simulink model "feng_ct"  (R2016b)
settings: Solver=VariableStepAuto  StartTime=0.0  StopTime=5000  RelTol=1e-3  EnableMultiTasking=on
undefined symbols (not defined in the file or in its folder): fft_stages, output_len_bits, xengbits
undefined symbols (not defined in the file): input_bits, total_bits, total_bits2
libraries: xbsIndex_r4 x10571, casper_library_misc x48, casper_library_scopes x9, xps_library x2
(part 11 of 81)

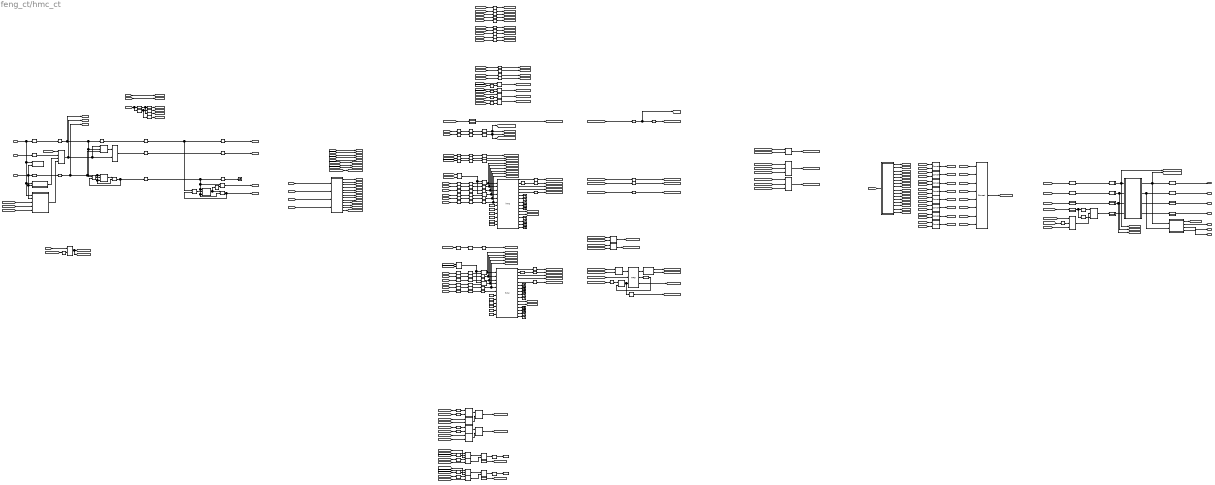
== system feng_ct/hmc_ct ==
  note: Double buffer the data to form output packets
  note: Eight parallel channels.
  note: TVG
  note: Write two successive words together.
  note: Sync debugging - did we get two syncs
      | so close we weren't even reading out yet?
  note: Check for _en sync and bank errors
  note: HMC
  in_sync : Inport
  in_dv : Inport  Port=2
  in_d128 : Inport  Port=3
  Assertion : Assertion
  Assertion1 : Assertion
  Concat{3..10,12} (9 alike) : xbsIndex_r4/Concat  num_inputs=2  dbl_ovrd=off  block_type=concat
  Concat11 : xbsIndex_r4/Concat  num_inputs=8  dbl_ovrd=off  block_type=concat
  Concat13 : xbsIndex_r4/Concat  num_inputs=3  dbl_ovrd=off  block_type=concat
  Constant{,3,6,9} (4 alike) : xbsIndex_r4/Constant  const=0  gui_display_data_type=Boolean  arith_type=Boolean  n_bits=16  bin_pt=14  preci_type=Single  exp_width=8  frac_width=24  explicit_period=on  period=1  equ=P=C  opselect=C  inp2=PCIN>>17  opr=+  inp1=P  carry=CIN  dbl_ovrd=off  block_type=constant
  Constant{1,4,7,10} (4 alike) : xbsIndex_r4/Constant  const=0  gui_display_data_type=Fixed-point  arith_type=Unsigned  n_bits=27  bin_pt=0  preci_type=Single  exp_width=8  frac_width=24  explicit_period=on  period=1  equ=P=C  opselect=C  inp2=PCIN>>17  opr=+  inp1=P  carry=CIN  dbl_ovrd=off  block_type=constant
  Constant11 : xbsIndex_r4/Constant  const=0  gui_display_data_type=Fixed-point  arith_type=Unsigned  n_bits=9  bin_pt=0  preci_type=Single  exp_width=8  frac_width=24  explicit_period=on  period=1  equ=P=C  opselect=C  inp2=PCIN>>17  opr=+  inp1=P  carry=CIN  dbl_ovrd=off  block_type=constant
  Constant12 : xbsIndex_r4/Constant  const=0  gui_display_data_type=Boolean  arith_type=Boolean  n_bits=9  bin_pt=0  preci_type=Single  exp_width=8  frac_width=24  explicit_period=on  period=1  equ=P=C  opselect=C  inp2=PCIN>>17  opr=+  inp1=P  carry=CIN  dbl_ovrd=off  block_type=constant
  Constant13 : xbsIndex_r4/Constant  const=0  gui_display_data_type=Boolean  arith_type=Boolean  n_bits=9  bin_pt=0  preci_type=Single  exp_width=8  frac_width=24  explicit_period=on  period=1  equ=P=C  opselect=C  inp2=PCIN>>17  opr=+  inp1=P  carry=CIN  dbl_ovrd=off  block_type=constant
  Constant2 : xbsIndex_r4/Constant  const=0  gui_display_data_type=Fixed-point  arith_type=Unsigned  n_bits=256  bin_pt=0  preci_type=Single  exp_width=8  frac_width=24  explicit_period=on  period=1  equ=P=C  opselect=C  inp2=PCIN>>17  opr=+  inp1=P  carry=CIN  dbl_ovrd=off  block_type=constant
  Constant5 : xbsIndex_r4/Constant  const=0  gui_display_data_type=Fixed-point  arith_type=Unsigned  n_bits=9  bin_pt=0  preci_type=Single  exp_width=8  frac_width=24  explicit_period=on  period=1  equ=P=C  opselect=C  inp2=PCIN>>17  opr=+  inp1=P  carry=CIN  dbl_ovrd=off  block_type=constant
  Constant8 : xbsIndex_r4/Constant  const=0  gui_display_data_type=Fixed-point  arith_type=Unsigned  n_bits=256  bin_pt=0  preci_type=Single  exp_width=8  frac_width=24  explicit_period=on  period=1  equ=P=C  opselect=C  inp2=PCIN>>17  opr=+  inp1=P  carry=CIN  dbl_ovrd=off  block_type=constant
  Delay{,1..2,4..13,16..19,21..23,25..27,30..32,41,43..50,52..53,56..58,61..62,66..69,72,74,76..92} (65 alike) : xbsIndex_r4/Delay  rst=off  infoeditControl=Selection of Reset will increase slice count due to use of real FFs and instead of SRLs  en=off  latency=1  reg_retiming=off  dbl_ovrd=off  block_type=delay
      settings: infoedit=Hardware notes: A delay line is a chain, each link of which is an SRL16 or SRL32 followed by a flip-flop.
  Delay{14..15,35,39,42,93} (6 alike) : xbsIndex_r4/Delay  rst=off  infoeditControl=Selection of Reset will increase slice count due to use of real FFs and instead of SRLs  en=off  latency=2  reg_retiming=off  dbl_ovrd=off  block_type=delay
      settings: infoedit=Hardware notes: A delay line is a chain, each link of which is an SRL16 or SRL32 followed by a flip-flop.
  Delay{3,20,24,28..29,37..38,40,55,59,63,70..71,73} (14 alike) : xbsIndex_r4/Delay  rst=off  infoeditControl=Selection of Reset will increase slice count due to use of real FFs and instead of SRLs  en=off  latency=5  reg_retiming=off  dbl_ovrd=off  block_type=delay
      settings: infoedit=Hardware notes: A delay line is a chain, each link of which is an SRL16 or SRL32 followed by a flip-flop.
  Delay33 : xbsIndex_r4/Delay  rst=off  infoeditControl=Selection of Reset will increase slice count due to use of real FFs and instead of SRLs  en=off  latency=4  reg_retiming=off  dbl_ovrd=off  block_type=delay
      settings: infoedit=Hardware notes: A delay line is a chain, each link of which is an SRL16 or SRL32 followed by a flip-flop.
  Delay34 : xbsIndex_r4/Delay  rst=off  infoeditControl=Selection of Reset will increase slice count due to use of real FFs and instead of SRLs  en=off  latency=4  reg_retiming=off  dbl_ovrd=off  block_type=delay
      settings: infoedit=Hardware notes: A delay line is a chain, each link of which is an SRL16 or SRL32 followed by a flip-flop.
  Delay36 : xbsIndex_r4/Delay  rst=off  infoeditControl=Selection of Reset will increase slice count due to use of real FFs and instead of SRLs  en=off  latency=4  reg_retiming=off  dbl_ovrd=off  block_type=delay
      settings: infoedit=Hardware notes: A delay line is a chain, each link of which is an SRL16 or SRL32 followed by a flip-flop.
  Inverter{,1..11,15..16} (14 alike) : xbsIndex_r4/Inverter  en=off  latency=0  dbl_ovrd=off  block_type=inv
  Logical{,3,8,19,21,29..31} (8 alike) : xbsIndex_r4/Logical  logical_function=AND  inputs=2  en=off  latency=0  precision=Full  arith_type=Unsigned  n_bits=16  bin_pt=0  align_bp=on  dbl_ovrd=off  block_type=logical
  Logical1 : xbsIndex_r4/Logical  logical_function=AND  inputs=2  en=off  latency=1  precision=User Defined  arith_type=Boolean  n_bits=1  bin_pt=0  align_bp=on  dbl_ovrd=off  block_type=logical
  Logical{2,9..10,20} (4 alike) : xbsIndex_r4/Logical  logical_function=OR  inputs=2  en=off  latency=0  precision=Full  arith_type=Unsigned  n_bits=16  bin_pt=0  align_bp=on  dbl_ovrd=off  block_type=logical
  Logical{5,7,11,13,17..18,22,28} (8 alike) : xbsIndex_r4/Logical  logical_function=AND  inputs=2  en=off  latency=5  precision=Full  arith_type=Unsigned  n_bits=16  bin_pt=0  align_bp=on  dbl_ovrd=off  block_type=logical
  Logical{4,12,16,26} (4 alike) : xbsIndex_r4/Logical  logical_function=AND  inputs=2  en=off  latency=1  precision=Full  arith_type=Unsigned  n_bits=16  bin_pt=0  align_bp=on  dbl_ovrd=off  block_type=logical
  Logical14 : xbsIndex_r4/Logical  logical_function=OR  inputs=2  en=off  latency=5  precision=Full  arith_type=Unsigned  n_bits=16  bin_pt=0  align_bp=on  dbl_ovrd=off  block_type=logical
  Logical15 : xbsIndex_r4/Logical  logical_function=AND  inputs=2  en=off  latency=2  precision=Full  arith_type=Unsigned  n_bits=16  bin_pt=0  align_bp=on  dbl_ovrd=off  block_type=logical
  Logical23 : xbsIndex_r4/Logical  logical_function=OR  inputs=2  en=off  latency=5  precision=Full  arith_type=Unsigned  n_bits=16  bin_pt=0  align_bp=on  dbl_ovrd=off  block_type=logical
  Logical24 : xbsIndex_r4/Logical  logical_function=AND  inputs=3  en=off  latency=5  precision=Full  arith_type=Unsigned  n_bits=16  bin_pt=0  align_bp=on  dbl_ovrd=off  block_type=logical
  Logical25 : xbsIndex_r4/Logical  logical_function=AND  inputs=2  en=off  latency=1  precision=User Defined  arith_type=Boolean  n_bits=1  bin_pt=0  align_bp=on  dbl_ovrd=off  block_type=logical
  Logical32 : xbsIndex_r4/Logical  logical_function=OR  inputs=2  en=off  latency=2  precision=Full  arith_type=Unsigned  n_bits=16  bin_pt=0  align_bp=on  dbl_ovrd=off  block_type=logical
  Logical6 : xbsIndex_r4/Logical  logical_function=AND  inputs=3  en=off  latency=5  precision=Full  arith_type=Unsigned  n_bits=16  bin_pt=0  align_bp=on  dbl_ovrd=off  block_type=logical
  Mux : xbsIndex_r4/Mux  inputs=2  en=off  latency=2  precision=Full  arith_type=Unsigned  n_bits=16  bin_pt=14  quantization=Truncate  overflow=Wrap  dbl_ovrd=off  block_type=mux
  Mux1 : xbsIndex_r4/Mux  inputs=2  en=off  latency=2  precision=Full  arith_type=Unsigned  n_bits=16  bin_pt=14  quantization=Truncate  overflow=Wrap  dbl_ovrd=off  block_type=mux
  Mux2 : xbsIndex_r4/Mux  inputs=2  en=off  latency=2  precision=Full  arith_type=Unsigned  n_bits=16  bin_pt=14  quantization=Truncate  overflow=Wrap  dbl_ovrd=off  block_type=mux
  Mux3 : xbsIndex_r4/Mux  inputs=3  en=off  latency=2  precision=Full  arith_type=Unsigned  n_bits=16  bin_pt=14  quantization=Truncate  overflow=Wrap  dbl_ovrd=off  block_type=mux
  Register : xbsIndex_r4/Register  init=0  rst=on  en=on  dbl_ovrd=off  block_type=register
  Register1 : xbsIndex_r4/Register  init=0  rst=on  en=on  dbl_ovrd=off  block_type=register
  Slice{8..9,12..13} (4 alike) : xbsIndex_r4/Slice  nbits=1  boolean_output=on  mode=Lower Bit Location + Width  bit1=0  base1=MSB of Input  bit0=input_len_bits - 2 + output_len_bits  base0=LSB of Input  dbl_ovrd=off  block_type=slice
  Terminator{,1..18} (19 alike) : Terminator
  bank2 : xbsIndex_r4/Slice  nbits=12  boolean_output=off  mode=Upper Bit Location + Width  bit1=-4  base1=MSB of Input  bit0=128  base0=LSB of Input  dbl_ovrd=off  block_type=slice
  bank3 : xbsIndex_r4/Slice  nbits=12  boolean_output=off  mode=Upper Bit Location + Width  bit1=-4  base1=MSB of Input  bit0=128  base0=LSB of Input  dbl_ovrd=off  block_type=slice
  bank4 : xbsIndex_r4/Slice  nbits=128  boolean_output=off  mode=Lower Bit Location + Width  bit1=0  base1=MSB of Input  bit0=128  base0=LSB of Input  dbl_ovrd=off  block_type=slice
  bank5 : xbsIndex_r4/Slice  nbits=128  boolean_output=off  mode=Lower Bit Location + Width  bit1=0  base1=MSB of Input  bit0=0  base0=LSB of Input  dbl_ovrd=off  block_type=slice
  bank6 : xbsIndex_r4/Slice  nbits=12  boolean_output=on  mode=Upper Bit Location + Width  bit1=0  base1=MSB of Input  bit0=128  base0=LSB of Input  dbl_ovrd=off  block_type=slice
  bank7 : xbsIndex_r4/Slice  nbits=12  boolean_output=on  mode=Upper Bit Location + Width  bit1=0  base1=MSB of Input  bit0=128  base0=LSB of Input  dbl_ovrd=off  block_type=slice
  bus_create1 : Subsystem  AncestorBlock=casper_library_flow_control/bus_create  mask(bus_create){inputNum=2}
      mask prompts: inputNum "Number of inputs:"
      mask init:
      | bus_create_init(gcb,...
      |     'inputNum', inputNum);
  bus_expand1 : Subsystem  AncestorBlock=casper_library_flow_control/bus_expand  mask(bus_expand){mode=divisions of equal size, outputNum=16, outputWidth=16, outputBinaryPt=0, outputArithmeticType=0, show_format=off, outputToWorkspace=off, variablePrefix=out, outputToModelAsWell=on}
      mask prompts: outputNum "Number of outputs:"; outputWidth "Output width:"; outputBinaryPt "Output binary point position:"; outputArithmeticType "Output arithmetic type (ufix=0, fix=1, bool=2):"; show_format "Print format string?"; outputToWorkspace "Output to workspace?"; variablePrefix "Variable name prefix:"; outputToModelAsWell "Output to model as well?"
      mask help:
      | Expands a 'bus' made using a bus_create or Xilinx
      | concat block.
      | The input will be divided into the specified number
      | of outputs with the specified arithmetic types.
      | Divisions are made from most significant bit.
      mask init: same as feng_ct/bus_expand1
      settings: AttributesFormatString=16 outputs
      mask TypeOptions mode: divisions of equal size | divisions of arbitrary size
      mask Callback mode: bus_expand_callback();
      mask Callback outputWidth: bus_expand_callback();
      mask Callback outputToWorkspace: bus_expand_callback();
  bus_expand2 : Subsystem  AncestorBlock=casper_library_flow_control/bus_expand  mask(bus_expand){mode=divisions of arbitrary size, outputNum=1, outputWidth=[256 9], outputBinaryPt=0, outputArithmeticType=0, show_format=on, outputToWorkspace=off, variablePrefix=out, outputToModelAsWell=on}
      mask prompts: outputNum "Number of outputs:"; outputWidth "Output width [msb ... lsb]:"; outputBinaryPt "Output binary point position [msb ... lsb]:"; outputArithmeticType "Output arithmetic type (ufix=0, fix=1, bool=2) [msb ... lsb]:"; show_format "Print format string?"; outputToWorkspace "Output to workspace?"; variablePrefix "Variable name prefix:"; outputToModelAsWell "Output to model as well?"
      mask help:
      | Expands a 'bus' made using a bus_create or Xilinx
      | concat block.
      | The input will be divided into the specified number
      | of outputs with the specified arithmetic types.
      | Divisions are made from most significant bit.
      mask init: same as feng_ct/bus_expand1
      settings: AttributesFormatString=2 outputs: uf256.0,uf9.0,
      mask TypeOptions mode: divisions of equal size | divisions of arbitrary size
      mask Callback mode: bus_expand_callback();
      mask Callback outputWidth: bus_expand_callback();
      mask Callback outputToWorkspace: bus_expand_callback();
  convert_rd_en1 : xbsIndex_r4/Convert  gui_display_data_type=Boolean  arith_type=Boolean  n_bits=128  bin_pt=0  float_type=Single  exp_bits=8  fraction_bits=24  quantization=Truncate  overflow=Wrap  en=off  latency=0  pipeline=off  dbl_ovrd=off  block_type=convert
      settings: xl_area=[0, 0, 0, 0, 0, 0, 0]
  convert_rd_en4 : xbsIndex_r4/Convert  gui_display_data_type=Boolean  arith_type=Boolean  n_bits=128  bin_pt=0  float_type=Single  exp_bits=8  fraction_bits=24  quantization=Truncate  overflow=Wrap  en=off  latency=0  pipeline=off  dbl_ovrd=off  block_type=convert
      settings: xl_area=[0, 0, 0, 0, 0, 0, 0]
  d1_fifo : xbsIndex_r4/FIFO  mem_type=Distributed RAM  performance_options=Standard_FIFO  embedded_registers=off  depth=16  percent_nbits=1  rst=off  rst_latency=1  en=off  use_dcount=off  use_percent_full_port=off  use_almost_empty=off  almost_empty_thresh=2  use_almost_full=off  almost_full_thresh=14  explicit_period=off  dbl_ovrd=off  block_type=fifo
  edge_detect1 : Subsystem  AncestorBlock=casper_library_misc/edge_detect  mask(edge_detect){edge=Rising, polarity=Active High, x_in=[0 0.08 0.08 0.16 0.16 0.24 0.24 0.32 0.32 0.4], y_in=[-1 -1  1  1  1  1  1  1  1  1], x_out=[0.6 0.68 0.68 0.76 0.76 0.84 0.84 0.92 0.92 1], y_out=[-1 -1  1  1 -1 -1 -1 -1 -1 -1]}
      mask prompts: edge "Edge Type"; polarity "Output Polarity"; x_in "Input X Positions"; y_in "Input Y Positions"; x_out "Output X Positions"; y_out "Output Y Positions"
      mask help: Output is active for one-cycle after each edge of the specified type (i.e. rising, falling or both).
      mask init: same as feng_ct/edge_detect1
      settings: AttributesFormatString=|
      | rising edges
      | active high
      mask Help: Output is active for one-cycle after each edge of the specified type (i.e. rising, falling, or both).  Latency is zero.
      mask TypeOptions edge: Rising | Falling | Both
      mask TypeOptions polarity: Active High | Active Low
      mask Display:
      | plot(x_in_num,0.5+y_in_num*0.2);
      | plot(x_out_num,0.5+y_out_num*0.2);
  gen_freq_calc : Subsystem  mask{pkt_len_bits=5, lat=3}
      mask prompts: pkt_len_bits "Packet length bits"; lat "Latency"
      mask init:
      | display_string = sprintf('latency=%i', 7 * lat);
      | set_param(gcb, 'AttributesFormatString', display_string);
      settings: AttributesFormatString=latency=21
  hmc : xps_library/hmc  Tag=xps:hmc  mez=0  sim_depth=(input_len_bits-1) + output_len_bits + 1  sim_latency=5  sim_rand=on
  hmc1 : xps_library/hmc  Tag=xps:hmc  mez=1  sim_depth=(input_len_bits-1) + output_len_bits + 1  sim_latency=5  sim_rand=on
  hmc_addr_gen : Subsystem  mask{input_len_bits=input_len_bits - 1}
      mask prompts: input_len_bits "Input vector bits"
  obuf : Subsystem  mask{output_vec_bits=output_len_bits, pkt_buffer_latency=10, omux_latency=15}
      mask prompts: output_vec_bits "CT output vector bits"; pkt_buffer_latency "Output buffer latency"; omux_latency "Output mux latency"
  prev_word : xbsIndex_r4/Register  init=0  rst=on  en=on  dbl_ovrd=off  block_type=register
  spectrum_ctr2 : xbsIndex_r4/Slice  nbits=256 - (32 + 9)  boolean_output=off  mode=Lower Bit Location + Width  bit1=-1  base1=MSB of Input  bit0=32 + 9  base0=LSB of Input  dbl_ovrd=off  block_type=slice
  spectrum_ctr3 : xbsIndex_r4/Slice  nbits=32  boolean_output=off  mode=Lower Bit Location + Width  bit1=-1  base1=MSB of Input  bit0=0  base0=LSB of Input  dbl_ovrd=off  block_type=slice
  spectrum_ctr4 : xbsIndex_r4/Slice  nbits=9  boolean_output=off  mode=Lower Bit Location + Width  bit1=-1  base1=MSB of Input  bit0=32  base0=LSB of Input  dbl_ovrd=off  block_type=slice
  tvg_data_gen : Subsystem
  tvg_data_gen_oneshot : Subsystem
      mask Display:
      | color('red');
      | disp('ONE SHOT!!');
      | % color('green');
      | % port_label('input', 1, 'dv')
      | % color('red');
      | % port_label('output', 1, 'err')
  tvg_data_tone_gen : Subsystem
  we_delay1 : Subsystem  AncestorBlock=casper_library_delays/pipeline  mask(pipeline){latency=2}
      mask help:
      | An explicitly laid-out delay line to avoid mapping to SRL16s
      | for use in pipelining to help achieve timing closure.
      mask init:
      | pipeline_init(gcb,'latency',latency);
      settings: AttributesFormatString=Latency = %<latency>
      mask Display:
      | port_label('input', 1, 'd');
      | port_label('output', 1, 'q');
      | disp(['Z^-', num2str(latency)]);
  we_delay10 : Subsystem  AncestorBlock=casper_library_delays/pipeline  mask(pipeline){latency=21}
      mask help:
      | An explicitly laid-out delay line to avoid mapping to SRL16s
      | for use in pipelining to help achieve timing closure.
      mask init:
      | pipeline_init(gcb,'latency',latency);
      settings: AttributesFormatString=Latency = %<latency>
      mask Display:
      | port_label('input', 1, 'd');
      | port_label('output', 1, 'q');
      | disp(['Z^-', num2str(latency)]);
  we_delay11 : Subsystem  AncestorBlock=casper_library_delays/pipeline  mask(pipeline){latency=2}
      mask help:
      | An explicitly laid-out delay line to avoid mapping to SRL16s
      | for use in pipelining to help achieve timing closure.
      mask init:
      | pipeline_init(gcb,'latency',latency);
      settings: AttributesFormatString=Latency = %<latency>
      mask Display:
      | port_label('input', 1, 'd');
      | port_label('output', 1, 'q');
      | disp(['Z^-', num2str(latency)]);
  we_delay12 : Subsystem  AncestorBlock=casper_library_delays/pipeline  mask(pipeline){latency=21}
      mask help:
      | An explicitly laid-out delay line to avoid mapping to SRL16s
      | for use in pipelining to help achieve timing closure.
      mask init:
      | pipeline_init(gcb,'latency',latency);
      settings: AttributesFormatString=Latency = %<latency>
      mask Display:
      | port_label('input', 1, 'd');
      | port_label('output', 1, 'q');
      | disp(['Z^-', num2str(latency)]);
  we_delay2 : Subsystem  AncestorBlock=casper_library_delays/pipeline  mask(pipeline){latency=2}
      mask help:
      | An explicitly laid-out delay line to avoid mapping to SRL16s
      | for use in pipelining to help achieve timing closure.
      mask init:
      | pipeline_init(gcb,'latency',latency);
      settings: AttributesFormatString=Latency = %<latency>
      mask Display:
      | port_label('input', 1, 'd');
      | port_label('output', 1, 'q');
      | disp(['Z^-', num2str(latency)]);
  we_delay3 : Subsystem  AncestorBlock=casper_library_delays/pipeline  mask(pipeline){latency=2}
      mask help:
      | An explicitly laid-out delay line to avoid mapping to SRL16s
      | for use in pipelining to help achieve timing closure.
      mask init:
      | pipeline_init(gcb,'latency',latency);
      settings: AttributesFormatString=Latency = %<latency>
      mask Display:
      | port_label('input', 1, 'd');
      | port_label('output', 1, 'q');
      | disp(['Z^-', num2str(latency)]);
  we_delay4 : Subsystem  AncestorBlock=casper_library_delays/pipeline  mask(pipeline){latency=2}
      mask help:
      | An explicitly laid-out delay line to avoid mapping to SRL16s
      | for use in pipelining to help achieve timing closure.
      mask init:
      | pipeline_init(gcb,'latency',latency);
      settings: AttributesFormatString=Latency = %<latency>
      mask Display:
      | port_label('input', 1, 'd');
      | port_label('output', 1, 'q');
      | disp(['Z^-', num2str(latency)]);
  we_delay5 : Subsystem  AncestorBlock=casper_library_delays/pipeline  mask(pipeline){latency=2}
      mask help:
      | An explicitly laid-out delay line to avoid mapping to SRL16s
      | for use in pipelining to help achieve timing closure.
      mask init:
      | pipeline_init(gcb,'latency',latency);
      settings: AttributesFormatString=Latency = %<latency>
      mask Display:
      | port_label('input', 1, 'd');
      | port_label('output', 1, 'q');
      | disp(['Z^-', num2str(latency)]);
  we_delay6 : Subsystem  AncestorBlock=casper_library_delays/pipeline  mask(pipeline){latency=2}
      mask help:
      | An explicitly laid-out delay line to avoid mapping to SRL16s
      | for use in pipelining to help achieve timing closure.
      mask init:
      | pipeline_init(gcb,'latency',latency);
      settings: AttributesFormatString=Latency = %<latency>
      mask Display:
      | port_label('input', 1, 'd');
      | port_label('output', 1, 'q');
      | disp(['Z^-', num2str(latency)]);
  we_delay7 : Subsystem  AncestorBlock=casper_library_delays/pipeline  mask(pipeline){latency=2}
      mask help:
      | An explicitly laid-out delay line to avoid mapping to SRL16s
      | for use in pipelining to help achieve timing closure.
      mask init:
      | pipeline_init(gcb,'latency',latency);
      settings: AttributesFormatString=Latency = %<latency>
      mask Display:
      | port_label('input', 1, 'd');
      | port_label('output', 1, 'q');
      | disp(['Z^-', num2str(latency)]);
  we_delay8 : Subsystem  AncestorBlock=casper_library_delays/pipeline  mask(pipeline){latency=21}
      mask help:
      | An explicitly laid-out delay line to avoid mapping to SRL16s
      | for use in pipelining to help achieve timing closure.
      mask init:
      | pipeline_init(gcb,'latency',latency);
      settings: AttributesFormatString=Latency = %<latency>
      mask Display:
      | port_label('input', 1, 'd');
      | port_label('output', 1, 'q');
      | disp(['Z^-', num2str(latency)]);
  we_delay9 : Subsystem  AncestorBlock=casper_library_delays/pipeline  mask(pipeline){latency=21}
      mask help:
      | An explicitly laid-out delay line to avoid mapping to SRL16s
      | for use in pipelining to help achieve timing closure.
      mask init:
      | pipeline_init(gcb,'latency',latency);
      settings: AttributesFormatString=Latency = %<latency>
      mask Display:
      | port_label('input', 1, 'd');
      | port_label('output', 1, 'q');
      | disp(['Z^-', num2str(latency)]);
  out_sync : Outport
  out_dv : Outport  Port=2
  out_d256 : Outport  Port=3
  pkt_start : Outport  Port=4
  freq_id : Outport  Port=5
  x_index : Outport  Port=6
  x_pkt_index : Outport  Port=7
  tag scope: ct_bank_error_g0=global, ct_bank_error_g1=global, ct_en_sync_error_g0=global, ct_en_sync_error_g1=global, ct_in_d0_g=global, ct_in_d0_msb_g=global, ct_in_d1_g=global, ct_in_d1_msb_g=global, ct_in_dv_g=global, ct_in_sync_g=global, cthmc_sync_err_g0=global, cthmc_sync_err_g1=global, hmc_d256_g0=global, hmc_d256_g1=global, hmc_dv_clash_g=global, hmc_dv_fixed_clash_g=global, hmc_dv_g0=global, hmc_dv_g1=global, hmc_err_rdrdy_g0=global, hmc_err_rdrdy_g1=global, hmc_err_wrrdy_g0=global, hmc_err_wrrdy_g1=global, hmc_fifo_full_g=global, hmc_init_done_g0=global, hmc_init_done_g1=global, hmc_postokay_g0=global, hmc_postokay_g1=global, hmc_rd_rdy_g0=global, hmc_rd_rdy_g1=global, hmc_sync_g=global, hmc_tag_g0=global, hmc_tag_g1=global, hmc_wr_rdy_g0=global, hmc_wr_rdy_g1=global, hmc_wr_sync_g0=global, hmc_wr_sync_g1=global, obuf_in_dv=global, obuf_in_sync=global, obuf_in_tag=global, qt_d128_g=global, qt_dv_g=global, qt_sync_g=global, raw_freq_ctr_g=global, rd_addr_final_g0=global, rd_addr_final_g1=global, rd_addr_raw_final_g0=global, rd_arm_final_g0=global, rd_arm_final_g1=global, rd_en_final_g0=global, rd_en_final_g1=global, rd_tag_final_g0=global, sync_hmc_in0=global, sync_hmc_in1=global, sync_obuf_in=global, sync_obuf_out=global, wr_addr_final_g0=global, wr_addr_final_g1=global, wr_addr_raw_g0=global, wr_data_final_g0=global, wr_data_final_g1=global, wr_en_final_g0=global, wr_en_final_g1=global
  wires:
  we_delay10/1(q) -> out_sync/1
  we_delay8/1(q) -> out_dv/1
  we_delay9/1(q) -> out_d256/1
  we_delay12/1(q) -> pkt_start/1
  we_delay3/1(q) -> we_delay4/1(d)
  we_delay2/1(q) -> we_delay5/1(d)
  we_delay1/1(q) -> we_delay6/1(d)
  we_delay11/1(q) -> spectrum_ctr2/1, spectrum_ctr3/1
  [hmc_sync] -> we_delay3/1(d)
  [hmc_dv] -> we_delay2/1(d)
  [hmc_tag] -> we_delay1/1(d)
  [hmc_d256_reo] -> we_delay11/1(d)
  [ct_tag_insert_sel] -> Mux/1
  [hmc_d256_reo] -> spectrum_ctr4/1
  spectrum_ctr4/1 -> Mux/2
  [hmc_tag] -> Mux/3
  we_delay7/1(q) -> obuf/4(in_d256)
  Concat13/1 -> we_delay7/1(d)
  spectrum_ctr3/1 -> Concat13/3
  Mux/1 -> Concat13/2
  spectrum_ctr2/1 -> Concat13/1
  Concat11/1 -> [hmc_d256_reo]
  we_delay6/1(q) -> obuf/3(in_tag), [obuf_in_tag]
  we_delay5/1(q) -> obuf/2(in_dv), [obuf_in_dv]
  we_delay4/1(q) -> obuf/1(in_sync), [obuf_in_sync], [sync_obuf_in]
  obuf/4(pkt_start) -> we_delay12/1(d)
  obuf/3(out_d) -> we_delay9/1(d)
  obuf/2(out_dv) -> gen_freq_calc/2(dv), we_delay8/1(d)
  obuf/1(out_sync) -> gen_freq_calc/1(sync), we_delay10/1(d), [sync_obuf_out]
  [dbuf7] -> Concat11/8
  [dbuf6] -> Concat11/7
  [dbuf5] -> Concat11/6
  [dbuf4] -> Concat11/5
  [dbuf3] -> Concat11/4
  [dbuf2] -> Concat11/3
  [dbuf0] -> Concat11/1
  [dbuf1] -> Concat11/2
  Concat10/1 -> [dbuf7]
  Concat12/1 -> [dbuf6]
  Concat9/1 -> [dbuf5]
  Concat8/1 -> [dbuf4]
  Concat7/1 -> [dbuf3]
  Concat6/1 -> [dbuf2]
  Concat5/1 -> [dbuf1]
  Concat4/1 -> [dbuf0]
  [p0f7] -> Concat10/1
  [p0f6] -> Concat12/1
  [p1f5] -> Concat9/2
  [p0f5] -> Concat9/1
  [p1f4] -> Concat8/2
  [p0f4] -> Concat8/1
  [p1f3] -> Concat7/2
  [p0f3] -> Concat7/1
  [p1f2] -> Concat6/2
  [p0f2] -> Concat6/1
  [p0f1] -> Concat5/1
  [p1f1] -> Concat5/2
  [p1f7] -> Concat10/2
  [p1f6] -> Concat12/2
  [p1f0] -> Concat4/2
  [p0f0] -> Concat4/1
  bus_expand1/16(lsb_out1) -> [p1f7]
  bus_expand1/15(out2) -> [p1f6]
  bus_expand1/14(out3) -> [p1f5]
  bus_expand1/13(out4) -> [p1f4]
  bus_expand1/12(out5) -> [p0f7]  "d256_f7"
  bus_expand1/11(out6) -> [p0f6]  "d256_f6"
  bus_expand1/10(out7) -> [p0f5]  "d256_f5"
  bus_expand1/9(out8) -> [p0f4]  "d256_f4"
  bus_expand1/8(out9) -> [p1f3]
  bus_expand1/7(out10) -> [p1f2]
  bus_expand1/6(out11) -> [p1f1]
  bus_expand1/5(out12) -> [p1f0]
  bus_expand1/4(out13) -> [p0f3]  "d256_f3"
  bus_expand1/3(out14) -> [p0f2]  "d256_f2"
  bus_expand1/2(out15) -> [p0f1]  "d256_f1"
  bus_expand1/1(msb_out16) -> [p0f0]  "d256_f0"
  [hmc_d256] -> bus_expand1/1(bus_in)
  Delay39/1 -> [qt_dv_g], Register/1, Register/3, Logical3/2, prev_word/3
  Delay35/1 -> [qt_sync_g], Delay1/1, prev_word/2, Logical2/1
  in_d128/1 -> Delay34/1
  [ct_tvg_en] -> Mux3/1
  Delay1/1 -> Delay15/1
  Logical3/1 -> Delay42/1, Logical2/2
  Register/1 -> Logical3/1
  Logical2/1 -> Register/2
  Concat3/1 -> Delay14/1
  Mux3/1 -> [qt_d128_g], prev_word/1, Concat3/2  "data128"
  prev_word/1 -> Concat3/1
  in_dv/1 -> tvg_data_gen_oneshot/2(dv), Delay33/1, tvg_data_gen/2(dv), tvg_data_tone_gen/2(dv)  "dv128"
  in_sync/1 -> tvg_data_gen_oneshot/1(sync), tvg_data_gen/1(sync), tvg_data_tone_gen/1(sync), Delay36/1  "sync128"
  [d256] -> bank5/1, bank4/1
  [dv256] -> [ct_in_dv_g]
  [sync256] -> [ct_in_sync_g]
  bank2/1 -> [ct_in_d0_g]
  bank4/1 -> bank6/1, bank2/1
  bank5/1 -> bank7/1, bank3/1
  bank3/1 -> [ct_in_d1_g]
  Delay33/1 -> Delay39/1
  Delay36/1 -> Delay35/1
  bank6/1 -> [ct_in_d0_msb_g]
  bank7/1 -> [ct_in_d1_msb_g]
  [rd_addr_arm_raw0] -> Inverter6/1
  [sync256] -> Logical15/1
  Inverter6/1 -> Logical15/2
  Logical15/1 -> [cthmc_sync_err_g1], [cthmc_sync_err_g0]
  [tvgtone_p0] -> tvg_data_tone_gen/3(target0)
  [tvgtone_p1] -> tvg_data_tone_gen/4(target1)
  [tvgtone_levels] -> tvg_data_tone_gen/5(levels)
  tvg_data_tone_gen/1(d128) -> Mux3/4
  Delay15/1 -> Delay44/1, Logical9/1  "sync256"
  Delay14/1 -> Delay43/1  "d256"
  Delay42/1 -> Logical12/2, Register1/3, Register1/1, Logical16/1, Delay45/1  "dv_256"
  Register1/1 -> Logical12/1, Inverter3/1  "this"
  Logical16/1 -> [dv256_0]  "ONE"
  Inverter3/1 -> Logical16/2
  Delay45/1 -> Terminator/1  "ORIG"
  Delay43/1 -> [d256]
  Logical12/1 -> [dv256_1], Logical9/2  "TWO"
  Logical9/1 -> Register1/2
  Delay44/1 -> [sync256]
  Delay34/1 -> Mux3/2
  tvg_data_gen/1(d128) -> Mux3/3
  [wr_addr_0] -> [wr_addr_1]
  [wr_d256_0] -> [wr_d256_1]
  [rd_addr_0] -> [rd_addr_1]
  [rd_tag_0] -> [rd_tag_1]
  [wr_sync_0] -> [wr_sync_1]
  [wr_addr_raw0] -> [wr_addr_raw1]
  [rd_addr_arm0] -> [rd_addr_arm1]
  [rd_addr_raw0] -> [rd_addr_raw1]
  [rd_addr_arm_raw0] -> [rd_addr_arm_raw1]
  [rd_arm_final_g0] -> Logical6/3
  Delay23/1 -> Delay12/1
  Delay22/1 -> Delay11/1
  Delay21/1 -> Delay9/1
  Delay10/1 -> Delay4/1
  Delay7/1 -> Delay5/1
  [wr_addr_0] -> Delay7/1
  Delay6/1 -> Delay2/1
  Delay4/1 -> Delay40/1  "WR_sync"
  [wr_sync_0] -> Delay10/1
  Delay3/1 -> [wr_addr_raw_g0]
  Delay2/1 -> Delay3/1  "WR_raw_addr"
  [wr_addr_raw0] -> Delay6/1
  Logical13/1 -> Logical14/2  "RD_SE_ERR"
  Inverter2/1 -> Assertion/1  "SE_ERR"
  Logical14/1 -> Inverter2/1
  Logical6/1 -> Logical14/1  "WR_SE_ERR"
  Inverter5/1 -> Logical13/1
  [rd_en_final_g0] -> Logical13/2
  [wr_en_final_g0] -> Inverter5/1
  Inverter/1 -> Logical6/2
  [rd_en_final_g0] -> Inverter/1
  [wr_en_final_g0] -> Logical6/1
  [rd_tag_0] -> Delay23/1
  [rd_addr_0] -> Delay22/1
  [rd_en_0] -> Delay21/1
  Delay12/1 -> Delay38/1  "RD_tag"
  Delay5/1 -> Delay20/1  "WR_addr"
  Delay8/1 -> Delay24/1
  Delay11/1 -> Delay37/1  "RD_rdaddr"
  Delay17/1 -> Delay13/1
  Delay18/1 -> Delay8/1
  Logical5/1 -> hmc/1, [wr_en_final_g0]
  Delay13/1 -> Logical5/2  "WR_en"
  Logical11/1 -> hmc/4, [rd_en_final_g0]
  Delay9/1 -> Logical11/2  "RD_en"
  Delay24/1 -> hmc/3, [wr_data_final_g0]
  Delay37/1 -> hmc/5, [rd_addr_final_g0]
  Delay38/1 -> hmc/6, [rd_tag_final_g0]
  [init_done0] -> Logical7/1
  [postokay0] -> Logical7/2
  [wr_en_final_g0] -> Logical1/1
  Inverter4/1 -> Logical1/2
  Logical1/1 -> [hmc_err_wrrdy_g0]  "err_wrrdy"
  [hmc_wr_rdy_0] -> Inverter4/1
  Inverter1/1 -> Logical4/2
  [rd_en_final_g0] -> Logical4/1
  [hmc_rd_rdy_0] -> Inverter1/1
  Logical4/1 -> [hmc_err_rdrdy_g0]
  [init_done1] -> Delay19/1
  [postokay1] -> Delay41/1
  Delay19/1 -> [hmc_init_done_g1]
  Delay41/1 -> [hmc_postokay_g1]
  [wr_en_0] -> Delay17/1
  [wr_d256_0] -> Delay18/1
  [wr_addr_final_g0] -> Slice12/1
  [rd_addr_final_g0] -> Slice13/1
  Slice13/1 -> Logical/2  "final_rd_bank"
  Slice12/1 -> Logical/1  "final_wr_bank"
  Logical/1 -> Logical8/1
  Logical10/1 -> Logical8/2
  [wr_en_final_g0] -> Logical10/1
  [rd_en_final_g0] -> Logical10/2
  Logical8/1 -> [ct_bank_error_g0]  "same_bank"
  hmc/12 -> [postokay0]
  hmc/11 -> [init_done0]
  hmc/5 -> Delay31/1
  hmc/4 -> [hmc_rd_rdy_0]
  hmc/3 -> [hmc_wr_rdy_0]
  convert_rd_en4/1 -> Delay30/1  "hmcout_dv"
  Delay31/1 -> [hmc_tag_0_tmp]  "hmc_tag"
  Delay30/1 -> [hmc_dv_0_tmp]  "hmc_dv"
  Delay32/1 -> [hmc_d256_0_tmp]
  hmc/1 -> Delay32/1  "hmc_d256"
  hmc/2 -> convert_rd_en4/1
  Delay40/1 -> [hmc_wr_sync_g0], [sync_hmc_in0]
  [rd_addr_arm0] -> edge_detect1/1(in)
  edge_detect1/1(out) -> [hmc_sync_tmp]
  Logical7/1 -> Logical11/1, Logical5/1
  Delay29/1 -> [rd_addr_raw_final_g0]
  Delay28/1 -> [rd_arm_final_g0]
  Delay27/1 -> Delay28/1
  Delay26/1 -> Delay27/1
  [rd_addr_arm0] -> Delay26/1
  Delay25/1 -> Delay16/1
  Delay16/1 -> Delay29/1  "RD_raw_addr"
  [rd_addr_raw0] -> Delay25/1
  Delay20/1 -> [wr_addr_final_g0], hmc/2
  [wr_addr_final_g1] -> Slice8/1
  [rd_addr_final_g1] -> Slice9/1
  Slice9/1 -> Logical19/2  "final_rd_bank"
  Slice8/1 -> Logical19/1  "final_wr_bank"
  Logical19/1 -> Logical21/1
  Logical20/1 -> Logical21/2
  [wr_en_final_g1] -> Logical20/1
  [rd_en_final_g1] -> Logical20/2
  Logical21/1 -> [ct_bank_error_g1]  "same_bank"
  [rd_arm_final_g1] -> Logical24/3
  Logical22/1 -> Logical23/2  "RD_SE_ERR"
  Inverter8/1 -> Assertion1/1  "SE_ERR"
  Logical23/1 -> Inverter8/1
  Logical24/1 -> Logical23/1  "WR_SE_ERR"
  Inverter9/1 -> Logical22/1
  [rd_en_final_g1] -> Logical22/2
  [wr_en_final_g1] -> Inverter9/1
  Inverter7/1 -> Logical24/2
  [rd_en_final_g1] -> Inverter7/1
  [wr_en_final_g1] -> Logical24/1
  [wr_en_final_g1] -> Logical25/1
  Inverter11/1 -> Logical25/2
  Logical25/1 -> [hmc_err_wrrdy_g1]  "err_wrrdy"
  [hmc_wr_rdy_1] -> Inverter11/1
  Inverter10/1 -> Logical26/2
  [rd_en_final_g1] -> Logical26/1
  [hmc_rd_rdy_1] -> Inverter10/1
  Logical26/1 -> [hmc_err_rdrdy_g1]
  Delay66/1 -> Delay72/1
  Delay72/1 -> Delay73/1  "WR_sync"
  [wr_sync_1] -> Delay66/1
  Delay73/1 -> [sync_hmc_in1], [hmc_wr_sync_g1]
  [hmc_d256_0] -> Delay79/1
  [hmc_wr_rdy_0] -> Delay77/1
  [hmc_rd_rdy_0] -> Delay78/1
  [hmc_dv_0] -> Delay80/1
  [hmc_tag_0] -> Delay81/1
  [hmc_wr_rdy_1] -> Delay82/1
  [hmc_rd_rdy_1] -> Delay83/1
  [hmc_d256_1] -> Delay84/1
  [hmc_dv_1] -> Delay85/1
  [hmc_tag_1] -> Delay86/1
  Delay77/1 -> [hmc_wr_rdy_g0]
  Delay78/1 -> [hmc_rd_rdy_g0]
  Delay79/1 -> [hmc_d256_g0]
  Delay80/1 -> [hmc_dv_g0]
  Delay81/1 -> [hmc_tag_g0]
  Delay82/1 -> [hmc_wr_rdy_g1]
  Delay83/1 -> [hmc_rd_rdy_g1]
  Delay84/1 -> [hmc_d256_g1]
  Delay85/1 -> [hmc_dv_g1]
  Delay86/1 -> [hmc_tag_g1]
  Constant/1 -> hmc/7
  Constant1/1 -> hmc/8
  Constant2/1 -> hmc/9
  Constant3/1 -> hmc/10
  Constant4/1 -> hmc/11
  Constant5/1 -> hmc/12
  hmc/7 -> Terminator2/1
  hmc/6 -> Terminator1/1
  hmc/8 -> Terminator3/1
  hmc/9 -> Terminator4/1
  hmc/10 -> Terminator5/1
  hmc/13 -> Terminator6/1
  hmc/14 -> Terminator7/1
  hmc/15 -> Terminator8/1
  hmc/16 -> Terminator9/1
  [init_done0] -> Delay46/1
  [postokay0] -> Delay47/1
  Delay46/1 -> [hmc_init_done_g0]
  Delay47/1 -> [hmc_postokay_g0]
  Delay58/1 -> Delay49/1
  Delay57/1 -> Delay48/1
  Delay56/1 -> Delay88/1
  Delay76/1 -> Delay74/1
  [wr_addr_1] -> Delay76/1
  [rd_tag_1] -> Delay58/1
  [rd_addr_1] -> Delay57/1
  [rd_en_1] -> Delay56/1
  Delay49/1 -> Delay71/1  "RD_tag"
  Delay74/1 -> Delay55/1  "WR_addr"
  Delay87/1 -> Delay59/1
  Delay48/1 -> Delay70/1  "RD_rdaddr"
  Delay52/1 -> Delay50/1
  Delay53/1 -> Delay87/1
  Logical18/1 -> [wr_en_final_g1], hmc1/1
  Delay50/1 -> Logical18/2  "WR_en"
  Logical17/1 -> [rd_en_final_g1], hmc1/4
  Delay88/1 -> Logical17/2  "RD_en"
  Delay59/1 -> [wr_data_final_g1], hmc1/3
  Delay70/1 -> [rd_addr_final_g1], hmc1/5
  Delay71/1 -> hmc1/6
  [init_done1] -> Logical28/1
  [postokay1] -> Logical28/2
  [wr_en_1] -> Delay52/1
  [wr_d256_1] -> Delay53/1
  hmc1/12 -> [postokay1]
  hmc1/11 -> [init_done1]
  hmc1/5 -> Delay68/1
  hmc1/4 -> [hmc_rd_rdy_1]
  hmc1/3 -> [hmc_wr_rdy_1]
  convert_rd_en1/1 -> Delay67/1  "hmcout_dv"
  Delay68/1 -> [hmc_tag_1_tmp]  "hmc_tag"
  Delay67/1 -> [hmc_dv_1_tmp]  "hmc_dv"
  Delay69/1 -> [hmc_d256_1_tmp]
  hmc1/1 -> Delay69/1  "hmc_d256"
  hmc1/2 -> convert_rd_en1/1
  Logical28/1 -> Logical18/1, Logical17/1
  Delay63/1 -> [rd_arm_final_g1]
  Delay62/1 -> Delay63/1
  Delay61/1 -> Delay62/1
  [rd_addr_arm1] -> Delay61/1
  Delay55/1 -> hmc1/2, [wr_addr_final_g1]
  Constant6/1 -> hmc1/7
  Constant7/1 -> hmc1/8
  Constant8/1 -> hmc1/9
  Constant9/1 -> hmc1/10
  Constant10/1 -> hmc1/11
  Constant11/1 -> hmc1/12
  hmc1/7 -> Terminator11/1
  hmc1/6 -> Terminator10/1
  hmc1/8 -> Terminator12/1
  hmc1/9 -> Terminator13/1
  hmc1/10 -> Terminator14/1
  hmc1/13 -> Terminator15/1
  hmc1/14 -> Terminator16/1
  hmc1/15 -> Terminator17/1
  hmc1/16 -> Terminator18/1
  [sync256] -> hmc_addr_gen/1(sync)
  [dv256_1] -> hmc_addr_gen/4(dv1)
  [d256] -> hmc_addr_gen/2(d256)
  hmc_addr_gen/3(wr_en1) -> [wr_en_1]
  hmc_addr_gen/4(wr_addr) -> [wr_addr_0]
  hmc_addr_gen/5(wr_d256) -> [wr_d256_0]
  hmc_addr_gen/6(rd_en0) -> [rd_en_0]
  hmc_addr_gen/8(rd_addr) -> [rd_addr_0]
  hmc_addr_gen/9(rd_tag) -> [rd_tag_0]
  hmc_addr_gen/1(wr_sync) -> [wr_sync_0]
  hmc_addr_gen/10(wr_addr_raw) -> [wr_addr_raw0]
  hmc_addr_gen/11(rd_addr_arm) -> [rd_addr_arm0]
  hmc_addr_gen/12(rd_addr_raw) -> [rd_addr_raw0]
  hmc_addr_gen/13(rd_arm_raw) -> [rd_addr_arm_raw0]
  [dv256_0] -> hmc_addr_gen/3(dv0)
  hmc_addr_gen/2(wr_en0) -> [wr_en_0]
  hmc_addr_gen/7(rd_en1) -> [rd_en_1]
  [hmc_sync_tmp] -> Delay89/1
  Delay89/1 -> [hmc_sync_g], Delay93/1
  [hmc_d256_0_tmp] -> Delay90/1
  Delay90/1 -> [hmc_d256_0]
  [hmc_dv_0_tmp] -> Delay91/1
  Delay91/1 -> [hmc_dv_0]
  [hmc_tag_0_tmp] -> Delay92/1
  Delay92/1 -> [hmc_tag_0]
  bus_create1/1(bus_out) -> d1_fifo/1
  [hmc_d256_1_tmp] -> bus_create1/1(in1)
  [hmc_tag_1_tmp] -> bus_create1/2(in2)
  [hmc_dv_1_tmp] -> d1_fifo/2
  d1_fifo/2 -> Inverter15/1
  Logical30/1 -> Delay/1, d1_fifo/3
  Inverter15/1 -> Logical30/2
  [hmc_dv_0_tmp] -> Inverter16/1
  Inverter16/1 -> Logical30/1
  d1_fifo/1 -> bus_expand2/1(bus_in)
  bus_expand2/1(msb_out2) -> [hmc_d256_1]
  bus_expand2/2(lsb_out1) -> [hmc_tag_1]
  Delay/1 -> [hmc_dv_1]
  d1_fifo/3 -> [hmc_fifo_full_g]
  [hmc_dv_0_tmp] -> Logical29/1
  [hmc_dv_1_tmp] -> Logical29/2
  Logical29/1 -> [hmc_dv_clash_g]
  [hmc_dv_0] -> Logical31/1
  [hmc_dv_1] -> Logical31/2
  Logical31/1 -> [hmc_dv_fixed_clash_g]
  [hmc_dv_0] -> Mux1/1
  [hmc_tag_0] -> Mux1/3
  [hmc_tag_1] -> Mux1/2
  Mux1/1 -> [hmc_tag]
  [hmc_dv_0] -> Mux2/1
  [hmc_d256_0] -> Mux2/3
  [hmc_d256_1] -> Mux2/2
  Mux2/1 -> [hmc_d256]
  [hmc_dv_0] -> Logical32/1
  [hmc_dv_1] -> Logical32/2
  Logical32/1 -> [hmc_dv]
  Delay93/1 -> [hmc_sync]
  Constant12/1 -> [ct_en_sync_error_g0]
  Constant13/1 -> [ct_en_sync_error_g1]
  gen_freq_calc/1(raw_ctr64) -> [raw_freq_ctr_g]
  gen_freq_calc/2(freq) -> freq_id/1
  gen_freq_calc/3(x_index) -> x_index/1
  gen_freq_calc/4(x_pkt_index) -> x_pkt_index/1
